simulink model "Formation2CDOB"  (R2021a)
settings: Solver=VariableStepAuto  StartTime=0.0  StopTime=10  RelTol=1e-3
values from neighbouring files (symbols this model uses):
  alpha = param(2)    [DSR.m]    (also in DSRWithDelayPyra.m = param(1); DSR_ActDelay.m; NetConfigDSR.m = param(1); simulink_param.m = 1.912)
  delay = tau_a    (= 0.0077)    [StdConsPDDelay.m]    (also in simulink_param.m = 0.5)
  gnet = 40    [CDOB.m]    (also in StdConsPDDelay.m = 100; simulink_param.m = 0)
libraries: simulink x2
settings Model: Creator=shiva  LastModifiedBy=shiva

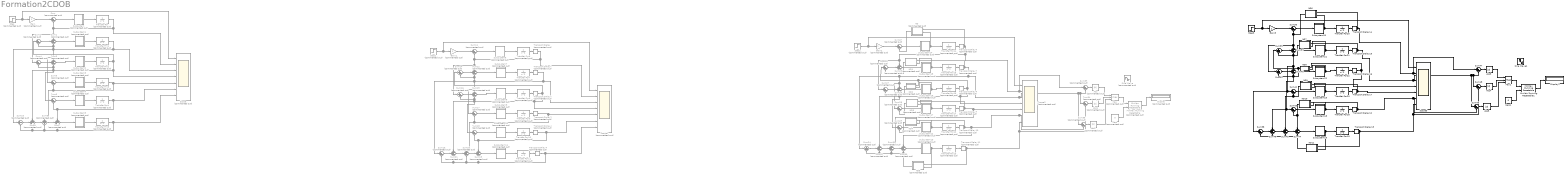
== system Formation2CDOB ==
  Abs : Abs  Commented=on
  Abs1 : Abs  Commented=on
  Abs2 : Abs  Commented=on
  Abs3 : Abs
  Abs4 : Abs
  Abs5 : Abs
  Display : Display  Commented=on
  Display1 : Display
  Gain : Gain  Commented=on
  Gain1 : Gain  Commented=on
  Gain2 : Gain  Commented=on
  Gain3 : Gain
  Max : MinMax  Commented=on  Function=max  Inputs=3
  Max1 : MinMax  Function=max  Inputs=3
  MinMax Running Resettable : simulink/Math Operations/MinMax Running Resettable  Commented=on  Function=max  vinit=0.0
  MinMax Running Resettable1 : simulink/Math Operations/MinMax Running Resettable  Function=max  vinit=0.0
  ND : Subsystem  Commented=on
  ND1 : Subsystem  Commented=on
  ND10 : Subsystem
  ND11 : Subsystem
  ND2 : Subsystem  Commented=on
  ND3 : Subsystem  Commented=on
  ND4 : Subsystem  Commented=on
  ND5 : Subsystem  Commented=on
  ND6 : Subsystem
  ND7 : Subsystem
  ND8 : Subsystem
  ND9 : Subsystem
  Scope : Scope  Commented=on  NumInputPorts=7
  Scope1 : Scope  Commented=on  NumInputPorts=7
  Scope2 : Scope  Commented=on  NumInputPorts=7
  Scope3 : Scope  NumInputPorts=7
  Sine Wave : Sin  Commented=on  SampleTime=0
  Sine Wave1 : Sin  SampleTime=0
  Step : Step  Commented=on  SampleTime=0
  Step1 : Step  Commented=on  SampleTime=0
  Step2 : Step  Commented=on  Time=0  After=10  SampleTime=0
  Step3 : Step  Time=0  After=10  SampleTime=0
  Subsystem : Subsystem  Commented=on
  Subsystem1 : Subsystem  Commented=on
  Subsystem10 : Subsystem  Commented=on
  Subsystem11 : Subsystem  Commented=on
  Subsystem12 : Subsystem  Commented=on
  Subsystem13 : Subsystem  Commented=on
  Subsystem14 : Subsystem  Commented=on
  Subsystem15 : Subsystem  Commented=on
  Subsystem16 : Subsystem  Commented=on
  Subsystem17 : Subsystem  Commented=on
  Subsystem18 : Subsystem
  Subsystem19 : Subsystem
  Subsystem2 : Subsystem  Commented=on
  Subsystem20 : Subsystem
  Subsystem21 : Subsystem
  Subsystem22 : Subsystem
  Subsystem23 : Subsystem
  Subsystem3 : Subsystem  Commented=on
  Subsystem4 : Subsystem  Commented=on
  Subsystem5 : Subsystem  Commented=on
  Subsystem6 : Subsystem  Commented=on
  Subsystem7 : Subsystem  Commented=on
  Subsystem8 : Subsystem  Commented=on
  Subsystem9 : Subsystem  Commented=on
  Sum{,2,4..6,10..11,13..14,16..18,22,24..25,27..29,33..35} (21 alike) : Sum  Commented=on  Inputs=|+-
  Sum{1,3,7..9,12,15,19..21,23,26,30..32} (15 alike) : Sum  Commented=on  Inputs=++-
  Sum{36,38..39,41..43,47..49} (9 alike) : Sum  Inputs=|+-
  Sum{37,40,44..46} (5 alike) : Sum  Inputs=++-
  Transfer Fcn{,1..17} (18 alike) : TransferFcn  Commented=on  Denominator=[1 0 0]
  Transfer Fcn{18..23} (6 alike) : TransferFcn  Denominator=[1 0 0]
  Transport Delay{,1..5} (6 alike) : TransportDelay  Commented=on  DelayTime=0.1
  Transport Delay{6..11} (6 alike) : TransportDelay  Commented=on  DelayTime=delay
  Transport Delay{12..17} (6 alike) : TransportDelay  DelayTime=delay
  Zero : Constant  Commented=on  Value=0  OutDataTypeStr=Inherit: Inherit via back propagation
  Zero1 : Constant  Value=0  OutDataTypeStr=Inherit: Inherit via back propagation
  wires:
  Subsystem/1(Out1) -> Transfer Fcn/1
  Subsystem1/1(Out1) -> Transfer Fcn1/1
  Subsystem2/1(Out1) -> Transfer Fcn2/1
  Subsystem3/1(Out1) -> Transfer Fcn3/1
  Subsystem4/1(Out1) -> Transfer Fcn4/1
  Subsystem5/1(Out1) -> Transfer Fcn5/1
  Step/1 -> Scope/1, Gain/1
  Sum/1 -> Subsystem/1(Input)
  Transfer Fcn/1 -> Scope/2, Sum1/1, Sum4/1, Sum/2
  Transfer Fcn1/1 -> Scope/3, Sum3/1, Sum5/1, Sum2/2, Sum1/3, Sum10/1
  Sum1/1 -> Subsystem1/1(Input)
  Sum2/1 -> Sum1/2
  Sum4/1 -> Sum3/2
  Transfer Fcn2/1 -> Scope/4, Sum6/1, Sum4/2, Sum3/3, Sum9/1, Sum2/1
  Sum3/1 -> Subsystem2/1(Input)
  Sum6/1 -> Subsystem4/1(Input)
  Sum5/1 -> Subsystem3/1(Input)
  Transfer Fcn3/1 -> Scope/5, Sum8/1, Sum5/2
  Transfer Fcn4/1 -> Scope/6, Sum7/1, Sum6/2
  Sum10/1 -> Sum9/2
  Sum9/1 -> Sum8/2
  Sum8/1 -> Sum7/2
  Sum7/1 -> Subsystem5/1(Input)
  Transfer Fcn5/1 -> Scope/7, Sum7/3, Sum8/3, Sum9/3, Sum10/2
  Gain/1 -> Sum/1
  Subsystem6/1(Out1) -> Transfer Fcn6/1
  Subsystem10/1(Out1) -> Transfer Fcn10/1
  Transfer Fcn11/1 -> Transport Delay5/1
  Sum14/1 -> Sum12/2
  Transfer Fcn10/1 -> Transport Delay4/1
  Transfer Fcn8/1 -> Transport Delay2/1
  Sum13/1 -> Sum21/2
  Subsystem7/1(Out1) -> Transfer Fcn7/1
  Sum18/1 -> Subsystem10/1(Input)
  Sum12/1 -> Subsystem7/1(Input)
  Step1/1 -> Scope1/1, Gain1/1
  Sum15/1 -> Subsystem8/1(Input)
  Gain1/1 -> Sum11/1
  Transfer Fcn6/1 -> Transport Delay/1
  Sum19/1 -> Subsystem11/1(Input)
  Subsystem9/1(Out1) -> Transfer Fcn9/1
  Subsystem8/1(Out1) -> Transfer Fcn8/1
  Sum21/1 -> Sum20/2
  Sum11/1 -> Subsystem6/1(Input)
  Sum17/1 -> Subsystem9/1(Input)
  Subsystem11/1(Out1) -> Transfer Fcn11/1
  Transfer Fcn9/1 -> Transport Delay3/1
  Transfer Fcn7/1 -> Transport Delay1/1
  Sum16/1 -> Sum15/2
  Sum20/1 -> Sum19/2
  Transport Delay/1 -> Sum12/1, Sum16/1, Sum11/2, Scope1/2
  Transport Delay1/1 -> Sum15/1, Sum17/1, Sum14/2, Sum12/3, Sum13/1, Scope1/3
  Transport Delay2/1 -> Scope1/4, Sum18/1, Sum16/2, Sum15/3, Sum21/1, Sum14/1
  Transport Delay3/1 -> Scope1/5, Sum20/1, Sum17/2
  Transport Delay4/1 -> Scope1/6, Sum19/1, Sum18/2
  Transport Delay5/1 -> Scope1/7, Sum19/3, Sum20/3, Sum21/3, Sum13/2
  Sum26/1 -> Subsystem16/1(Input)
  Gain2/1 -> Sum22/1
  Step2/1 -> Scope2/1, Gain2/1  "Reference"
  Subsystem15/1(Acc.) -> ND1/2(Acc.), Transfer Fcn15/1
  Transfer Fcn16/1 -> Transport Delay8/1
  Sum24/1 -> Sum32/2
  Sum23/1 -> Subsystem15/1(Input)
  Transfer Fcn12/1 -> Transport Delay10/1
  Transfer Fcn13/1 -> Transport Delay11/1
  Subsystem14/1(Acc.) -> ND/2(Acc.), Transfer Fcn14/1
  Transport Delay11/1 -> Scope2/7, Sum34/2, ND5/1(XRes)  "Agent 6"
  Sum31/1 -> Sum30/2
  Sum27/1 -> Sum26/2
  Sum25/1 -> Sum23/2
  Subsystem12/1(Acc.) -> ND4/2(Acc.), Transfer Fcn12/1
  Transfer Fcn17/1 -> Transport Delay9/1
  Sum29/1 -> Subsystem12/1(Input)
  Sum28/1 -> Subsystem17/1(Input)
  Subsystem13/1(Acc.) -> ND5/2(Acc.), Transfer Fcn13/1
  Sum22/1 -> Subsystem14/1(Input)
  Transfer Fcn15/1 -> Transport Delay7/1
  Sum30/1 -> Subsystem13/1(Input)
  Transfer Fcn14/1 -> Transport Delay6/1
  Subsystem16/1(Acc.) -> ND2/2(Acc.), Transfer Fcn16/1
  Transport Delay6/1 -> ND/1(XRes), Sum23/1, Sum27/1, Sum33/1, Scope2/2  "Agent 1"
  Transport Delay7/1 -> ND1/1(XRes), Sum26/1, Sum28/1, Sum24/1, Sum35/1, Sum34/1, Sum33/2, Scope2/3  "Agent 2"
  Transport Delay10/1 -> ND4/1(XRes), Sum35/2, Scope2/6, Sum30/1  "Agent 5"
  Subsystem17/1(Acc.) -> ND3/2(Acc.), Transfer Fcn17/1
  Transport Delay8/1 -> Scope2/4, Sum29/1, Sum32/1, ND2/1(XRes), Sum25/1  "Agent 3"
  Sum32/1 -> Sum31/2
  Transport Delay9/1 -> ND3/1(XRes), Scope2/5, Sum31/1  "Agent 4"
  ND/1(FeedBack) -> Sum22/2
  ND1/1(FeedBack) -> Sum25/2, Sum23/3
  ND2/1(FeedBack) -> Sum27/2, Sum26/3
  ND3/1(FeedBack) -> Sum28/2
  ND4/1(FeedBack) -> Sum29/2
  ND5/1(FeedBack) -> Sum24/2, Sum32/3, Sum31/3, Sum30/3
  Sum33/1 -> Abs/1
  Sum34/1 -> Abs1/1
  Abs/1 -> Max/1
  Abs1/1 -> Max/2
  Sum35/1 -> Abs2/1
  Abs2/1 -> Max/3
  MinMax Running Resettable/1 -> Display/1
  Zero/1 -> MinMax Running Resettable/2
  Max/1 -> MinMax Running Resettable/1
  Max1/1 -> MinMax Running Resettable1/1
  Abs3/1 -> Max1/1
  Sum49/1 -> Abs5/1
  Abs5/1 -> Max1/3
  MinMax Running Resettable1/1 -> Display1/1
  Sum47/1 -> Abs3/1
  Abs4/1 -> Max1/2
  Sum48/1 -> Abs4/1
  Sum41/1 -> Sum40/2
  ND8/1(FeedBack) -> Sum39/1, Sum41/2, Sum40/3, Sum46/1, Sum43/1
  Step3/1 -> Scope3/1, Gain3/1  "Reference"
  Transfer Fcn23/1 -> Transport Delay17/1
  Transport Delay12/1 -> ND10/1(XRes), Sum49/2, Scope3/6  "Agent 5"
  ND7/1(FeedBack) -> Sum39/2, Sum37/3, Sum40/1, Sum38/1, Sum42/1
  ND11/1(FeedBack) -> Sum38/2, Sum46/3, Sum45/3, Sum44/3
  ND10/1(FeedBack) -> Sum44/1, Sum43/2
  ND6/1(FeedBack) -> Sum41/1, Sum37/1, Sum36/2
  ND9/1(FeedBack) -> Sum45/1, Sum42/2
  Transport Delay17/1 -> ND9/1(XRes), Scope3/5  "Agent 4"
  Sum46/1 -> Sum45/2
  Transfer Fcn19/1 -> Transport Delay13/1
  Transport Delay15/1 -> ND7/1(XRes), Sum49/1, Sum48/1, Sum47/2, Scope3/3  "Agent 2"
  Transport Delay16/1 -> Scope3/4, ND8/1(XRes)  "Agent 3"
  Transport Delay14/1 -> ND6/1(XRes), Sum47/1, Scope3/2  "Agent 1"
  Subsystem23/1(Acc.) -> ND9/2(Acc.), Transfer Fcn23/1
  Subsystem20/1(Acc.) -> ND6/2(Acc.), Transfer Fcn20/1
  Sum36/1 -> Subsystem20/1(Input)
  Subsystem22/1(Acc.) -> ND8/2(Acc.), Transfer Fcn22/1
  Transfer Fcn20/1 -> Transport Delay14/1
  Subsystem19/1(Acc.) -> ND11/2(Acc.), Transfer Fcn19/1
  Sum37/1 -> Subsystem21/1(Input)
  Sum39/1 -> Sum37/2
  Transfer Fcn21/1 -> Transport Delay15/1
  Sum44/1 -> Subsystem19/1(Input)
  Sum42/1 -> Subsystem23/1(Input)
  Transport Delay13/1 -> Scope3/7, Sum48/2, ND11/1(XRes)  "Agent 6"
  Transfer Fcn22/1 -> Transport Delay16/1
  Sum38/1 -> Sum46/2
  Sum40/1 -> Subsystem22/1(Input)
  Sum45/1 -> Sum44/2
  Transfer Fcn18/1 -> Transport Delay12/1
  Sum43/1 -> Subsystem18/1(Input)
  Subsystem18/1(Acc.) -> ND10/2(Acc.), Transfer Fcn18/1
  Subsystem21/1(Acc.) -> ND7/2(Acc.), Transfer Fcn21/1
  Zero1/1 -> MinMax Running Resettable1/2
  Gain3/1 -> Sum36/1

== system Formation2CDOB/ND ==
  XRes : Inport
  Acc. : Inport  Port=2
  CDOB1 : Subsystem
  TimeDelayComp : Subsystem
  FeedBack : Outport
  wires:
  CDOB1/1(Dobsv) -> TimeDelayComp/2(Dobsv)
  Acc./1 -> CDOB1/2(Acc.)
  TimeDelayComp/1(FeedBack) -> FeedBack/1
  XRes/1 -> TimeDelayComp/1(SysOut), CDOB1/1(XRes)

== system Formation2CDOB/ND1 ==
  XRes : Inport
  Acc. : Inport  Port=2
  CDOB1 : Subsystem
  TimeDelayComp : Subsystem
  FeedBack : Outport
  wires:
  CDOB1/1(Dobsv) -> TimeDelayComp/2(Dobsv)
  Acc./1 -> CDOB1/2(Acc.)
  TimeDelayComp/1(FeedBack) -> FeedBack/1
  XRes/1 -> TimeDelayComp/1(SysOut), CDOB1/1(XRes)

== system Formation2CDOB/ND10 ==
  XRes : Inport
  Acc. : Inport  Port=2
  CDOB1 : Subsystem
  TimeDelayComp : Subsystem
  FeedBack : Outport
  wires:
  CDOB1/1(Dobsv) -> TimeDelayComp/2(Dobsv)
  Acc./1 -> CDOB1/2(Acc.)
  TimeDelayComp/1(FeedBack) -> FeedBack/1
  XRes/1 -> TimeDelayComp/1(SysOut), CDOB1/1(XRes)

== system Formation2CDOB/ND11 ==
  XRes : Inport
  Acc. : Inport  Port=2
  CDOB1 : Subsystem
  TimeDelayComp : Subsystem
  FeedBack : Outport
  wires:
  CDOB1/1(Dobsv) -> TimeDelayComp/2(Dobsv)
  Acc./1 -> CDOB1/2(Acc.)
  TimeDelayComp/1(FeedBack) -> FeedBack/1
  XRes/1 -> TimeDelayComp/1(SysOut), CDOB1/1(XRes)

== system Formation2CDOB/ND2 ==
  XRes : Inport
  Acc. : Inport  Port=2
  CDOB1 : Subsystem
  TimeDelayComp : Subsystem
  FeedBack : Outport
  wires:
  CDOB1/1(Dobsv) -> TimeDelayComp/2(Dobsv)
  Acc./1 -> CDOB1/2(Acc.)
  TimeDelayComp/1(FeedBack) -> FeedBack/1
  XRes/1 -> TimeDelayComp/1(SysOut), CDOB1/1(XRes)

== system Formation2CDOB/ND3 ==
  XRes : Inport
  Acc. : Inport  Port=2
  CDOB1 : Subsystem
  TimeDelayComp : Subsystem
  FeedBack : Outport
  wires:
  CDOB1/1(Dobsv) -> TimeDelayComp/2(Dobsv)
  Acc./1 -> CDOB1/2(Acc.)
  TimeDelayComp/1(FeedBack) -> FeedBack/1
  XRes/1 -> TimeDelayComp/1(SysOut), CDOB1/1(XRes)

== system Formation2CDOB/ND4 ==
  XRes : Inport
  Acc. : Inport  Port=2
  CDOB1 : Subsystem
  TimeDelayComp : Subsystem
  FeedBack : Outport
  wires:
  CDOB1/1(Dobsv) -> TimeDelayComp/2(Dobsv)
  Acc./1 -> CDOB1/2(Acc.)
  TimeDelayComp/1(FeedBack) -> FeedBack/1
  XRes/1 -> TimeDelayComp/1(SysOut), CDOB1/1(XRes)

== system Formation2CDOB/ND5 ==
  XRes : Inport
  Acc. : Inport  Port=2
  CDOB1 : Subsystem
  TimeDelayComp : Subsystem
  FeedBack : Outport
  wires:
  CDOB1/1(Dobsv) -> TimeDelayComp/2(Dobsv)
  Acc./1 -> CDOB1/2(Acc.)
  TimeDelayComp/1(FeedBack) -> FeedBack/1
  XRes/1 -> TimeDelayComp/1(SysOut), CDOB1/1(XRes)

== system Formation2CDOB/ND6 ==
  XRes : Inport
  Acc. : Inport  Port=2
  CDOB1 : Subsystem
  TimeDelayComp : Subsystem
  FeedBack : Outport
  wires:
  CDOB1/1(Dobsv) -> TimeDelayComp/2(Dobsv)
  Acc./1 -> CDOB1/2(Acc.)
  TimeDelayComp/1(FeedBack) -> FeedBack/1
  XRes/1 -> TimeDelayComp/1(SysOut), CDOB1/1(XRes)

== system Formation2CDOB/ND7 ==
  XRes : Inport
  Acc. : Inport  Port=2
  CDOB1 : Subsystem
  TimeDelayComp : Subsystem
  FeedBack : Outport
  wires:
  CDOB1/1(Dobsv) -> TimeDelayComp/2(Dobsv)
  Acc./1 -> CDOB1/2(Acc.)
  TimeDelayComp/1(FeedBack) -> FeedBack/1
  XRes/1 -> TimeDelayComp/1(SysOut), CDOB1/1(XRes)

== system Formation2CDOB/ND8 ==
  XRes : Inport
  Acc. : Inport  Port=2
  CDOB1 : Subsystem
  TimeDelayComp : Subsystem
  FeedBack : Outport
  wires:
  CDOB1/1(Dobsv) -> TimeDelayComp/2(Dobsv)
  Acc./1 -> CDOB1/2(Acc.)
  TimeDelayComp/1(FeedBack) -> FeedBack/1
  XRes/1 -> TimeDelayComp/1(SysOut), CDOB1/1(XRes)

== system Formation2CDOB/ND9 ==
  XRes : Inport
  Acc. : Inport  Port=2
  CDOB1 : Subsystem
  TimeDelayComp : Subsystem
  FeedBack : Outport
  wires:
  CDOB1/1(Dobsv) -> TimeDelayComp/2(Dobsv)
  Acc./1 -> CDOB1/2(Acc.)
  TimeDelayComp/1(FeedBack) -> FeedBack/1
  XRes/1 -> TimeDelayComp/1(SysOut), CDOB1/1(XRes)

== system Formation2CDOB/Subsystem ==
  Input : Inport
  Derivative : Derivative  CoefficientInTFapproximation=0
  Gain1 : Gain  Gain=alpha^2
  Gain2 : Gain  Gain=2*alpha
  Sum11 : Sum  Inputs=|++
  Out1 : Outport
  wires:
  Derivative/1 -> Gain2/1
  Gain2/1 -> Sum11/2
  Gain1/1 -> Sum11/1
  Sum11/1 -> Out1/1
  Input/1 -> Derivative/1, Gain1/1

== system Formation2CDOB/Subsystem1 ==
  Input : Inport
  Derivative : Derivative  CoefficientInTFapproximation=0
  Gain1 : Gain  Gain=alpha^2
  Gain2 : Gain  Gain=2*alpha
  Sum11 : Sum  Inputs=|++
  Out1 : Outport
  wires:
  Derivative/1 -> Gain2/1
  Gain2/1 -> Sum11/2
  Gain1/1 -> Sum11/1
  Sum11/1 -> Out1/1
  Input/1 -> Derivative/1, Gain1/1

== system Formation2CDOB/Subsystem10 ==
  Input : Inport
  Derivative : Derivative  CoefficientInTFapproximation=0
  Gain1 : Gain  Gain=alpha^2
  Gain2 : Gain  Gain=2*alpha
  Sum11 : Sum  Inputs=|++
  Out1 : Outport
  wires:
  Derivative/1 -> Gain2/1
  Gain2/1 -> Sum11/2
  Gain1/1 -> Sum11/1
  Sum11/1 -> Out1/1
  Input/1 -> Derivative/1, Gain1/1

== system Formation2CDOB/Subsystem11 ==
  Input : Inport
  Derivative : Derivative  CoefficientInTFapproximation=0
  Gain1 : Gain  Gain=alpha^2
  Gain2 : Gain  Gain=2*alpha
  Sum11 : Sum  Inputs=|++
  Out1 : Outport
  wires:
  Derivative/1 -> Gain2/1
  Gain2/1 -> Sum11/2
  Gain1/1 -> Sum11/1
  Sum11/1 -> Out1/1
  Input/1 -> Derivative/1, Gain1/1

== system Formation2CDOB/Subsystem12 ==
  Input : Inport
  Derivative : Derivative  CoefficientInTFapproximation=0
  Gain1 : Gain  Gain=alpha^2
  Gain2 : Gain  Gain=2*alpha
  Sum11 : Sum  Inputs=|++
  Acc. : Outport
  wires:
  Derivative/1 -> Gain2/1
  Gain2/1 -> Sum11/2
  Gain1/1 -> Sum11/1
  Sum11/1 -> Acc./1
  Input/1 -> Derivative/1, Gain1/1

== system Formation2CDOB/Subsystem13 ==
  Input : Inport
  Derivative : Derivative  CoefficientInTFapproximation=0
  Gain1 : Gain  Gain=alpha^2
  Gain2 : Gain  Gain=2*alpha
  Sum11 : Sum  Inputs=|++
  Acc. : Outport
  wires:
  Derivative/1 -> Gain2/1
  Gain2/1 -> Sum11/2
  Gain1/1 -> Sum11/1
  Sum11/1 -> Acc./1
  Input/1 -> Derivative/1, Gain1/1

== system Formation2CDOB/Subsystem14 ==
  Input : Inport
  Derivative : Derivative  CoefficientInTFapproximation=0
  Gain1 : Gain  Gain=alpha^2
  Gain2 : Gain  Gain=2*alpha
  Sum11 : Sum  Inputs=|++
  Acc. : Outport
  wires:
  Derivative/1 -> Gain2/1
  Gain2/1 -> Sum11/2
  Gain1/1 -> Sum11/1
  Sum11/1 -> Acc./1
  Input/1 -> Derivative/1, Gain1/1

== system Formation2CDOB/Subsystem15 ==
  Input : Inport
  Derivative : Derivative  CoefficientInTFapproximation=0
  Gain1 : Gain  Gain=alpha^2
  Gain2 : Gain  Gain=2*alpha
  Sum11 : Sum  Inputs=|++
  Acc. : Outport
  wires:
  Derivative/1 -> Gain2/1
  Gain2/1 -> Sum11/2
  Gain1/1 -> Sum11/1
  Sum11/1 -> Acc./1
  Input/1 -> Derivative/1, Gain1/1

== system Formation2CDOB/Subsystem16 ==
  Input : Inport
  Derivative : Derivative  CoefficientInTFapproximation=0
  Gain1 : Gain  Gain=alpha^2
  Gain2 : Gain  Gain=2*alpha
  Sum11 : Sum  Inputs=|++
  Acc. : Outport
  wires:
  Derivative/1 -> Gain2/1
  Gain2/1 -> Sum11/2
  Gain1/1 -> Sum11/1
  Sum11/1 -> Acc./1
  Input/1 -> Derivative/1, Gain1/1

== system Formation2CDOB/Subsystem17 ==
  Input : Inport
  Derivative : Derivative  CoefficientInTFapproximation=0
  Gain1 : Gain  Gain=alpha^2
  Gain2 : Gain  Gain=2*alpha
  Sum11 : Sum  Inputs=|++
  Acc. : Outport
  wires:
  Derivative/1 -> Gain2/1
  Gain2/1 -> Sum11/2
  Gain1/1 -> Sum11/1
  Sum11/1 -> Acc./1
  Input/1 -> Derivative/1, Gain1/1

== system Formation2CDOB/Subsystem18 ==
  Input : Inport
  Derivative : Derivative  CoefficientInTFapproximation=0
  Gain1 : Gain  Gain=alpha^2
  Gain2 : Gain  Gain=2*alpha
  Sum11 : Sum  Inputs=|++
  Acc. : Outport
  wires:
  Derivative/1 -> Gain2/1
  Gain2/1 -> Sum11/2
  Gain1/1 -> Sum11/1
  Sum11/1 -> Acc./1
  Input/1 -> Derivative/1, Gain1/1

== system Formation2CDOB/Subsystem19 ==
  Input : Inport
  Derivative : Derivative  CoefficientInTFapproximation=0
  Gain1 : Gain  Gain=alpha^2
  Gain2 : Gain  Gain=2*alpha
  Sum11 : Sum  Inputs=|++
  Acc. : Outport
  wires:
  Derivative/1 -> Gain2/1
  Gain2/1 -> Sum11/2
  Gain1/1 -> Sum11/1
  Sum11/1 -> Acc./1
  Input/1 -> Derivative/1, Gain1/1

== system Formation2CDOB/Subsystem2 ==
  Input : Inport
  Derivative : Derivative  CoefficientInTFapproximation=0
  Gain1 : Gain  Gain=alpha^2
  Gain2 : Gain  Gain=2*alpha
  Sum11 : Sum  Inputs=|++
  Out1 : Outport
  wires:
  Derivative/1 -> Gain2/1
  Gain2/1 -> Sum11/2
  Gain1/1 -> Sum11/1
  Sum11/1 -> Out1/1
  Input/1 -> Derivative/1, Gain1/1

== system Formation2CDOB/Subsystem20 ==
  Input : Inport
  Derivative : Derivative  CoefficientInTFapproximation=0
  Gain1 : Gain  Gain=alpha^2
  Gain2 : Gain  Gain=2*alpha
  Sum11 : Sum  Inputs=|++
  Acc. : Outport
  wires:
  Derivative/1 -> Gain2/1
  Gain2/1 -> Sum11/2
  Gain1/1 -> Sum11/1
  Sum11/1 -> Acc./1
  Input/1 -> Derivative/1, Gain1/1

== system Formation2CDOB/Subsystem21 ==
  Input : Inport
  Derivative : Derivative  CoefficientInTFapproximation=0
  Gain1 : Gain  Gain=alpha^2
  Gain2 : Gain  Gain=2*alpha
  Sum11 : Sum  Inputs=|++
  Acc. : Outport
  wires:
  Derivative/1 -> Gain2/1
  Gain2/1 -> Sum11/2
  Gain1/1 -> Sum11/1
  Sum11/1 -> Acc./1
  Input/1 -> Derivative/1, Gain1/1

== system Formation2CDOB/Subsystem22 ==
  Input : Inport
  Derivative : Derivative  CoefficientInTFapproximation=0
  Gain1 : Gain  Gain=alpha^2
  Gain2 : Gain  Gain=2*alpha
  Sum11 : Sum  Inputs=|++
  Acc. : Outport
  wires:
  Derivative/1 -> Gain2/1
  Gain2/1 -> Sum11/2
  Gain1/1 -> Sum11/1
  Sum11/1 -> Acc./1
  Input/1 -> Derivative/1, Gain1/1

== system Formation2CDOB/Subsystem23 ==
  Input : Inport
  Derivative : Derivative  CoefficientInTFapproximation=0
  Gain1 : Gain  Gain=alpha^2
  Gain2 : Gain  Gain=2*alpha
  Sum11 : Sum  Inputs=|++
  Acc. : Outport
  wires:
  Derivative/1 -> Gain2/1
  Gain2/1 -> Sum11/2
  Gain1/1 -> Sum11/1
  Sum11/1 -> Acc./1
  Input/1 -> Derivative/1, Gain1/1

== system Formation2CDOB/Subsystem3 ==
  Input : Inport
  Derivative : Derivative  CoefficientInTFapproximation=0
  Gain1 : Gain  Gain=alpha^2
  Gain2 : Gain  Gain=2*alpha
  Sum11 : Sum  Inputs=|++
  Out1 : Outport
  wires:
  Derivative/1 -> Gain2/1
  Gain2/1 -> Sum11/2
  Gain1/1 -> Sum11/1
  Sum11/1 -> Out1/1
  Input/1 -> Derivative/1, Gain1/1

== system Formation2CDOB/Subsystem4 ==
  Input : Inport
  Derivative : Derivative  CoefficientInTFapproximation=0
  Gain1 : Gain  Gain=alpha^2
  Gain2 : Gain  Gain=2*alpha
  Sum11 : Sum  Inputs=|++
  Out1 : Outport
  wires:
  Derivative/1 -> Gain2/1
  Gain2/1 -> Sum11/2
  Gain1/1 -> Sum11/1
  Sum11/1 -> Out1/1
  Input/1 -> Derivative/1, Gain1/1

== system Formation2CDOB/Subsystem5 ==
  Input : Inport
  Derivative : Derivative  CoefficientInTFapproximation=0
  Gain1 : Gain  Gain=alpha^2
  Gain2 : Gain  Gain=2*alpha
  Sum11 : Sum  Inputs=|++
  Out1 : Outport
  wires:
  Derivative/1 -> Gain2/1
  Gain2/1 -> Sum11/2
  Gain1/1 -> Sum11/1
  Sum11/1 -> Out1/1
  Input/1 -> Derivative/1, Gain1/1

== system Formation2CDOB/Subsystem6 ==
  Input : Inport
  Derivative : Derivative  CoefficientInTFapproximation=0
  Gain1 : Gain  Gain=alpha^2
  Gain2 : Gain  Gain=2*alpha
  Sum11 : Sum  Inputs=|++
  Out1 : Outport
  wires:
  Derivative/1 -> Gain2/1
  Gain2/1 -> Sum11/2
  Gain1/1 -> Sum11/1
  Sum11/1 -> Out1/1
  Input/1 -> Derivative/1, Gain1/1

== system Formation2CDOB/Subsystem7 ==
  Input : Inport
  Derivative : Derivative  CoefficientInTFapproximation=0
  Gain1 : Gain  Gain=alpha^2
  Gain2 : Gain  Gain=2*alpha
  Sum11 : Sum  Inputs=|++
  Out1 : Outport
  wires:
  Derivative/1 -> Gain2/1
  Gain2/1 -> Sum11/2
  Gain1/1 -> Sum11/1
  Sum11/1 -> Out1/1
  Input/1 -> Derivative/1, Gain1/1

== system Formation2CDOB/Subsystem8 ==
  Input : Inport
  Derivative : Derivative  CoefficientInTFapproximation=0
  Gain1 : Gain  Gain=alpha^2
  Gain2 : Gain  Gain=2*alpha
  Sum11 : Sum  Inputs=|++
  Out1 : Outport
  wires:
  Derivative/1 -> Gain2/1
  Gain2/1 -> Sum11/2
  Gain1/1 -> Sum11/1
  Sum11/1 -> Out1/1
  Input/1 -> Derivative/1, Gain1/1

== system Formation2CDOB/Subsystem9 ==
  Input : Inport
  Derivative : Derivative  CoefficientInTFapproximation=0
  Gain1 : Gain  Gain=alpha^2
  Gain2 : Gain  Gain=2*alpha
  Sum11 : Sum  Inputs=|++
  Out1 : Outport
  wires:
  Derivative/1 -> Gain2/1
  Gain2/1 -> Sum11/2
  Gain1/1 -> Sum11/1
  Sum11/1 -> Out1/1
  Input/1 -> Derivative/1, Gain1/1

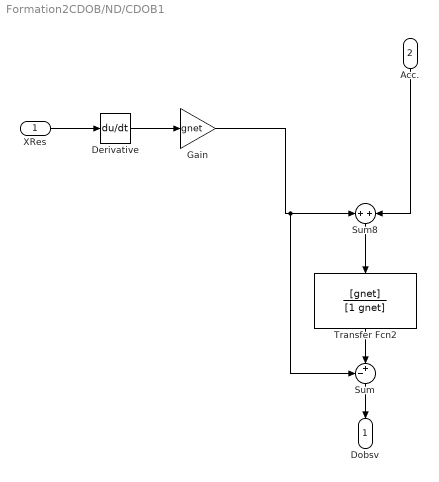
== system Formation2CDOB/ND/CDOB1 ==
  XRes : Inport
  Acc. : Inport  Port=2
  Derivative : Derivative  CoefficientInTFapproximation=0
  Gain : Gain  Gain=gnet
  Sum : Sum  Inputs=-+|
  Sum8 : Sum  Inputs=+|+
  Transfer Fcn2 : TransferFcn  Numerator=[gnet]  Denominator=[1 gnet]
  Dobsv : Outport
  wires:
  XRes/1 -> Derivative/1
  Acc./1 -> Sum8/2
  Transfer Fcn2/1 -> Sum/2
  Sum8/1 -> Transfer Fcn2/1
  Derivative/1 -> Gain/1
  Gain/1 -> Sum/1, Sum8/1
  Sum/1 -> Dobsv/1

== system Formation2CDOB/ND/TimeDelayComp ==
  SysOut : Inport
  Dobsv : Inport  Port=2
  DelayCom : TransferFcn  Denominator=[1 0 0]
  Sum8 : Sum  Inputs=|++
  FeedBack : Outport
  wires:
  DelayCom/1 -> Sum8/2
  SysOut/1 -> Sum8/1
  Sum8/1 -> FeedBack/1
  Dobsv/1 -> DelayCom/1

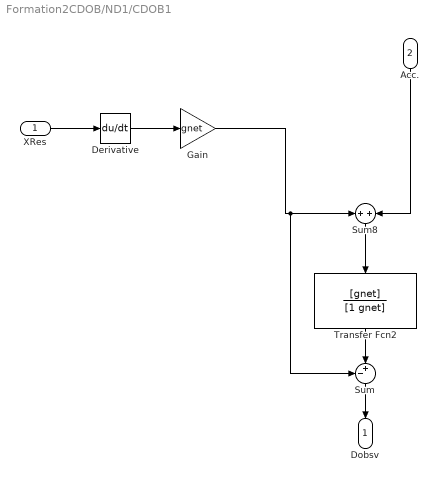
== system Formation2CDOB/ND1/CDOB1 ==
  XRes : Inport
  Acc. : Inport  Port=2
  Derivative : Derivative  CoefficientInTFapproximation=0
  Gain : Gain  Gain=gnet
  Sum : Sum  Inputs=-+|
  Sum8 : Sum  Inputs=+|+
  Transfer Fcn2 : TransferFcn  Numerator=[gnet]  Denominator=[1 gnet]
  Dobsv : Outport
  wires:
  XRes/1 -> Derivative/1
  Acc./1 -> Sum8/2
  Transfer Fcn2/1 -> Sum/2
  Sum8/1 -> Transfer Fcn2/1
  Derivative/1 -> Gain/1
  Gain/1 -> Sum/1, Sum8/1
  Sum/1 -> Dobsv/1

== system Formation2CDOB/ND1/TimeDelayComp ==
  SysOut : Inport
  Dobsv : Inport  Port=2
  DelayCom : TransferFcn  Denominator=[1 0 0]
  Sum8 : Sum  Inputs=|++
  FeedBack : Outport
  wires:
  DelayCom/1 -> Sum8/2
  SysOut/1 -> Sum8/1
  Sum8/1 -> FeedBack/1
  Dobsv/1 -> DelayCom/1

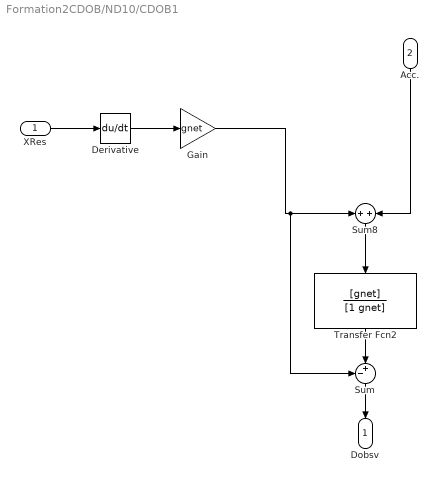
== system Formation2CDOB/ND10/CDOB1 ==
  XRes : Inport
  Acc. : Inport  Port=2
  Derivative : Derivative  CoefficientInTFapproximation=0
  Gain : Gain  Gain=gnet
  Sum : Sum  Inputs=-+|
  Sum8 : Sum  Inputs=+|+
  Transfer Fcn2 : TransferFcn  Numerator=[gnet]  Denominator=[1 gnet]
  Dobsv : Outport
  wires:
  XRes/1 -> Derivative/1
  Acc./1 -> Sum8/2
  Transfer Fcn2/1 -> Sum/2
  Sum8/1 -> Transfer Fcn2/1
  Derivative/1 -> Gain/1
  Gain/1 -> Sum/1, Sum8/1
  Sum/1 -> Dobsv/1

== system Formation2CDOB/ND10/TimeDelayComp ==
  SysOut : Inport
  Dobsv : Inport  Port=2
  DelayCom : TransferFcn  Denominator=[1 0 0]
  Sum8 : Sum  Inputs=|++
  FeedBack : Outport
  wires:
  DelayCom/1 -> Sum8/2
  SysOut/1 -> Sum8/1
  Sum8/1 -> FeedBack/1
  Dobsv/1 -> DelayCom/1

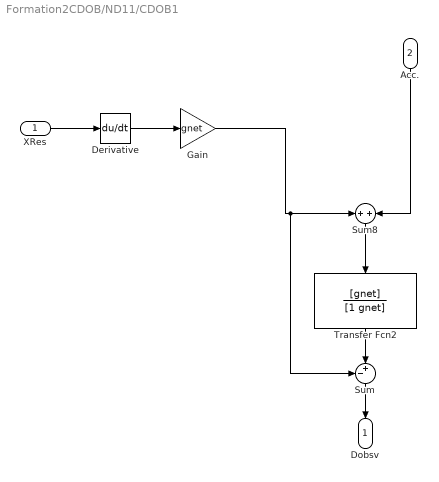
== system Formation2CDOB/ND11/CDOB1 ==
  XRes : Inport
  Acc. : Inport  Port=2
  Derivative : Derivative  CoefficientInTFapproximation=0
  Gain : Gain  Gain=gnet
  Sum : Sum  Inputs=-+|
  Sum8 : Sum  Inputs=+|+
  Transfer Fcn2 : TransferFcn  Numerator=[gnet]  Denominator=[1 gnet]
  Dobsv : Outport
  wires:
  XRes/1 -> Derivative/1
  Acc./1 -> Sum8/2
  Transfer Fcn2/1 -> Sum/2
  Sum8/1 -> Transfer Fcn2/1
  Derivative/1 -> Gain/1
  Gain/1 -> Sum/1, Sum8/1
  Sum/1 -> Dobsv/1

== system Formation2CDOB/ND11/TimeDelayComp ==
  SysOut : Inport
  Dobsv : Inport  Port=2
  DelayCom : TransferFcn  Denominator=[1 0 0]
  Sum8 : Sum  Inputs=|++
  FeedBack : Outport
  wires:
  DelayCom/1 -> Sum8/2
  SysOut/1 -> Sum8/1
  Sum8/1 -> FeedBack/1
  Dobsv/1 -> DelayCom/1

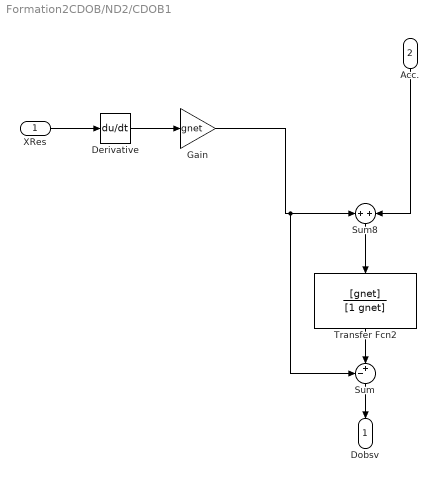
== system Formation2CDOB/ND2/CDOB1 ==
  XRes : Inport
  Acc. : Inport  Port=2
  Derivative : Derivative  CoefficientInTFapproximation=0
  Gain : Gain  Gain=gnet
  Sum : Sum  Inputs=-+|
  Sum8 : Sum  Inputs=+|+
  Transfer Fcn2 : TransferFcn  Numerator=[gnet]  Denominator=[1 gnet]
  Dobsv : Outport
  wires:
  XRes/1 -> Derivative/1
  Acc./1 -> Sum8/2
  Transfer Fcn2/1 -> Sum/2
  Sum8/1 -> Transfer Fcn2/1
  Derivative/1 -> Gain/1
  Gain/1 -> Sum/1, Sum8/1
  Sum/1 -> Dobsv/1

== system Formation2CDOB/ND2/TimeDelayComp ==
  SysOut : Inport
  Dobsv : Inport  Port=2
  DelayCom : TransferFcn  Denominator=[1 0 0]
  Sum8 : Sum  Inputs=|++
  FeedBack : Outport
  wires:
  DelayCom/1 -> Sum8/2
  SysOut/1 -> Sum8/1
  Sum8/1 -> FeedBack/1
  Dobsv/1 -> DelayCom/1

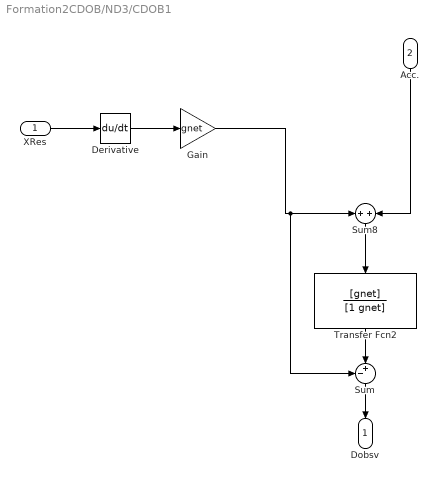
== system Formation2CDOB/ND3/CDOB1 ==
  XRes : Inport
  Acc. : Inport  Port=2
  Derivative : Derivative  CoefficientInTFapproximation=0
  Gain : Gain  Gain=gnet
  Sum : Sum  Inputs=-+|
  Sum8 : Sum  Inputs=+|+
  Transfer Fcn2 : TransferFcn  Numerator=[gnet]  Denominator=[1 gnet]
  Dobsv : Outport
  wires:
  XRes/1 -> Derivative/1
  Acc./1 -> Sum8/2
  Transfer Fcn2/1 -> Sum/2
  Sum8/1 -> Transfer Fcn2/1
  Derivative/1 -> Gain/1
  Gain/1 -> Sum/1, Sum8/1
  Sum/1 -> Dobsv/1

== system Formation2CDOB/ND3/TimeDelayComp ==
  SysOut : Inport
  Dobsv : Inport  Port=2
  DelayCom : TransferFcn  Denominator=[1 0 0]
  Sum8 : Sum  Inputs=|++
  FeedBack : Outport
  wires:
  DelayCom/1 -> Sum8/2
  SysOut/1 -> Sum8/1
  Sum8/1 -> FeedBack/1
  Dobsv/1 -> DelayCom/1

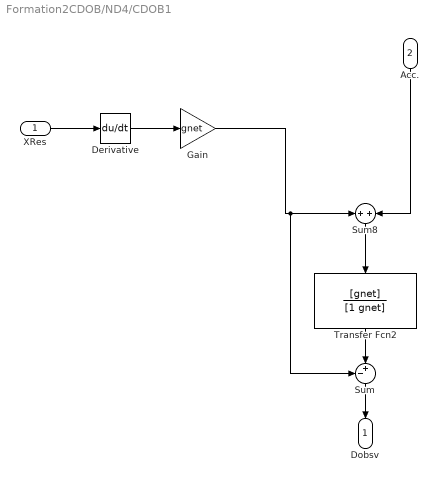
== system Formation2CDOB/ND4/CDOB1 ==
  XRes : Inport
  Acc. : Inport  Port=2
  Derivative : Derivative  CoefficientInTFapproximation=0
  Gain : Gain  Gain=gnet
  Sum : Sum  Inputs=-+|
  Sum8 : Sum  Inputs=+|+
  Transfer Fcn2 : TransferFcn  Numerator=[gnet]  Denominator=[1 gnet]
  Dobsv : Outport
  wires:
  XRes/1 -> Derivative/1
  Acc./1 -> Sum8/2
  Transfer Fcn2/1 -> Sum/2
  Sum8/1 -> Transfer Fcn2/1
  Derivative/1 -> Gain/1
  Gain/1 -> Sum/1, Sum8/1
  Sum/1 -> Dobsv/1

== system Formation2CDOB/ND4/TimeDelayComp ==
  SysOut : Inport
  Dobsv : Inport  Port=2
  DelayCom : TransferFcn  Denominator=[1 0 0]
  Sum8 : Sum  Inputs=|++
  FeedBack : Outport
  wires:
  DelayCom/1 -> Sum8/2
  SysOut/1 -> Sum8/1
  Sum8/1 -> FeedBack/1
  Dobsv/1 -> DelayCom/1

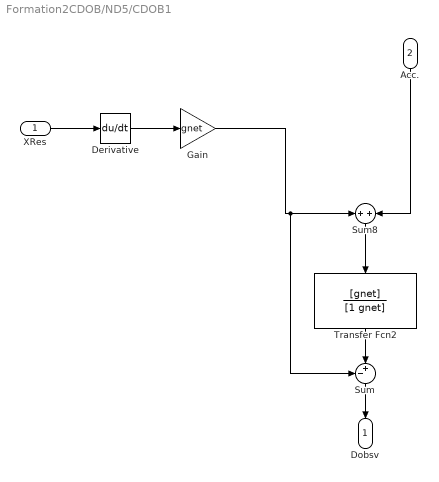
== system Formation2CDOB/ND5/CDOB1 ==
  XRes : Inport
  Acc. : Inport  Port=2
  Derivative : Derivative  CoefficientInTFapproximation=0
  Gain : Gain  Gain=gnet
  Sum : Sum  Inputs=-+|
  Sum8 : Sum  Inputs=+|+
  Transfer Fcn2 : TransferFcn  Numerator=[gnet]  Denominator=[1 gnet]
  Dobsv : Outport
  wires:
  XRes/1 -> Derivative/1
  Acc./1 -> Sum8/2
  Transfer Fcn2/1 -> Sum/2
  Sum8/1 -> Transfer Fcn2/1
  Derivative/1 -> Gain/1
  Gain/1 -> Sum/1, Sum8/1
  Sum/1 -> Dobsv/1

== system Formation2CDOB/ND5/TimeDelayComp ==
  SysOut : Inport
  Dobsv : Inport  Port=2
  DelayCom : TransferFcn  Denominator=[1 0 0]
  Sum8 : Sum  Inputs=|++
  FeedBack : Outport
  wires:
  DelayCom/1 -> Sum8/2
  SysOut/1 -> Sum8/1
  Sum8/1 -> FeedBack/1
  Dobsv/1 -> DelayCom/1

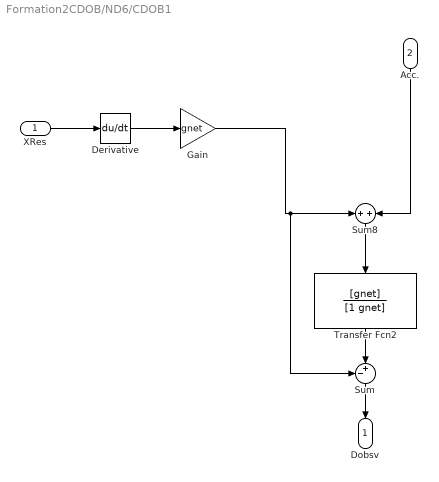
== system Formation2CDOB/ND6/CDOB1 ==
  XRes : Inport
  Acc. : Inport  Port=2
  Derivative : Derivative  CoefficientInTFapproximation=0
  Gain : Gain  Gain=gnet
  Sum : Sum  Inputs=-+|
  Sum8 : Sum  Inputs=+|+
  Transfer Fcn2 : TransferFcn  Numerator=[gnet]  Denominator=[1 gnet]
  Dobsv : Outport
  wires:
  XRes/1 -> Derivative/1
  Acc./1 -> Sum8/2
  Transfer Fcn2/1 -> Sum/2
  Sum8/1 -> Transfer Fcn2/1
  Derivative/1 -> Gain/1
  Gain/1 -> Sum/1, Sum8/1
  Sum/1 -> Dobsv/1

== system Formation2CDOB/ND6/TimeDelayComp ==
  SysOut : Inport
  Dobsv : Inport  Port=2
  DelayCom : TransferFcn  Denominator=[1 0 0]
  Sum8 : Sum  Inputs=|++
  FeedBack : Outport
  wires:
  DelayCom/1 -> Sum8/2
  SysOut/1 -> Sum8/1
  Sum8/1 -> FeedBack/1
  Dobsv/1 -> DelayCom/1

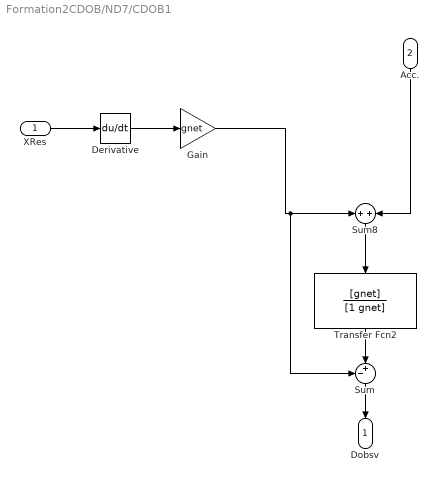
== system Formation2CDOB/ND7/CDOB1 ==
  XRes : Inport
  Acc. : Inport  Port=2
  Derivative : Derivative  CoefficientInTFapproximation=0
  Gain : Gain  Gain=gnet
  Sum : Sum  Inputs=-+|
  Sum8 : Sum  Inputs=+|+
  Transfer Fcn2 : TransferFcn  Numerator=[gnet]  Denominator=[1 gnet]
  Dobsv : Outport
  wires:
  XRes/1 -> Derivative/1
  Acc./1 -> Sum8/2
  Transfer Fcn2/1 -> Sum/2
  Sum8/1 -> Transfer Fcn2/1
  Derivative/1 -> Gain/1
  Gain/1 -> Sum/1, Sum8/1
  Sum/1 -> Dobsv/1

== system Formation2CDOB/ND7/TimeDelayComp ==
  SysOut : Inport
  Dobsv : Inport  Port=2
  DelayCom : TransferFcn  Denominator=[1 0 0]
  Sum8 : Sum  Inputs=|++
  FeedBack : Outport
  wires:
  DelayCom/1 -> Sum8/2
  SysOut/1 -> Sum8/1
  Sum8/1 -> FeedBack/1
  Dobsv/1 -> DelayCom/1

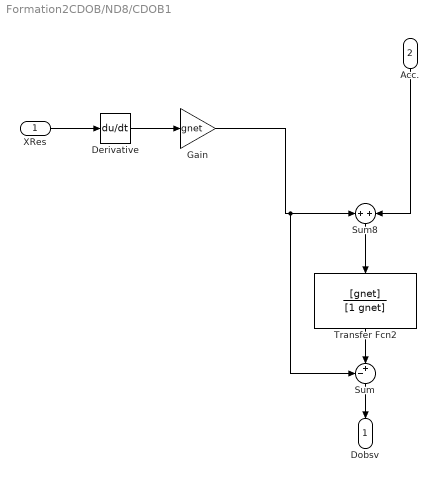
== system Formation2CDOB/ND8/CDOB1 ==
  XRes : Inport
  Acc. : Inport  Port=2
  Derivative : Derivative  CoefficientInTFapproximation=0
  Gain : Gain  Gain=gnet
  Sum : Sum  Inputs=-+|
  Sum8 : Sum  Inputs=+|+
  Transfer Fcn2 : TransferFcn  Numerator=[gnet]  Denominator=[1 gnet]
  Dobsv : Outport
  wires:
  XRes/1 -> Derivative/1
  Acc./1 -> Sum8/2
  Transfer Fcn2/1 -> Sum/2
  Sum8/1 -> Transfer Fcn2/1
  Derivative/1 -> Gain/1
  Gain/1 -> Sum/1, Sum8/1
  Sum/1 -> Dobsv/1

== system Formation2CDOB/ND8/TimeDelayComp ==
  SysOut : Inport
  Dobsv : Inport  Port=2
  DelayCom : TransferFcn  Denominator=[1 0 0]
  Sum8 : Sum  Inputs=|++
  FeedBack : Outport
  wires:
  DelayCom/1 -> Sum8/2
  SysOut/1 -> Sum8/1
  Sum8/1 -> FeedBack/1
  Dobsv/1 -> DelayCom/1

== system Formation2CDOB/ND9/CDOB1 ==
  XRes : Inport
  Acc. : Inport  Port=2
  Derivative : Derivative  CoefficientInTFapproximation=0
  Gain : Gain  Gain=gnet
  Sum : Sum  Inputs=-+|
  Sum8 : Sum  Inputs=+|+
  Transfer Fcn2 : TransferFcn  Numerator=[gnet]  Denominator=[1 gnet]
  Dobsv : Outport
  wires:
  XRes/1 -> Derivative/1
  Acc./1 -> Sum8/2
  Transfer Fcn2/1 -> Sum/2
  Sum8/1 -> Transfer Fcn2/1
  Derivative/1 -> Gain/1
  Gain/1 -> Sum/1, Sum8/1
  Sum/1 -> Dobsv/1

== system Formation2CDOB/ND9/TimeDelayComp ==
  SysOut : Inport
  Dobsv : Inport  Port=2
  DelayCom : TransferFcn  Denominator=[1 0 0]
  Sum8 : Sum  Inputs=|++
  FeedBack : Outport
  wires:
  DelayCom/1 -> Sum8/2
  SysOut/1 -> Sum8/1
  Sum8/1 -> FeedBack/1
  Dobsv/1 -> DelayCom/1
